simulink model "Torque_Control_ETR07"  (R2017b)
settings: Solver=FixedStepAuto  StartTime=0.0  StopTime=10.0  RelTol=1e-3
libraries: simulink x15
(part 3 of 5)

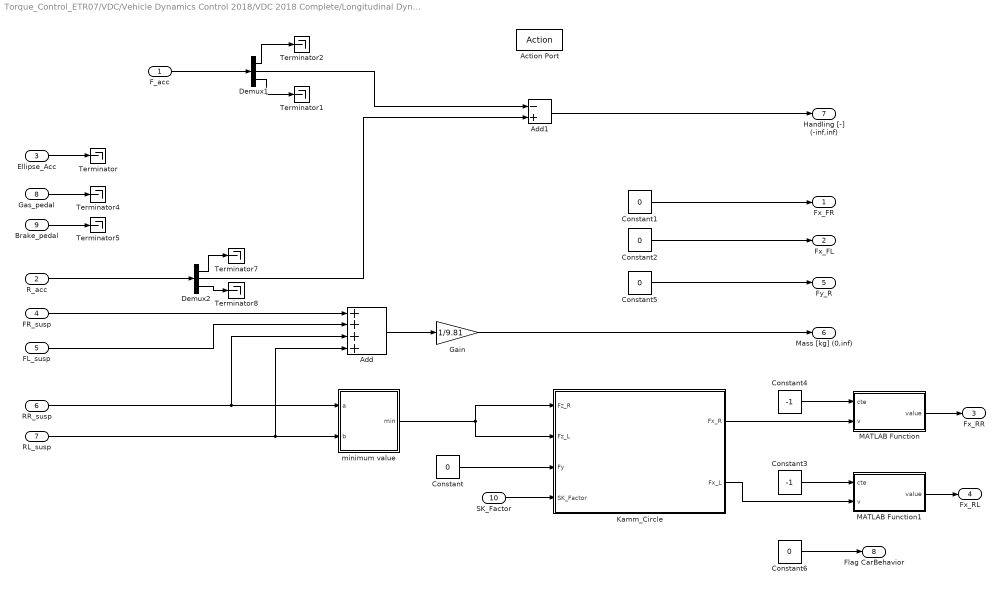
== system Torque_Control_ETR07/VDC/Vehicle Dynamics Control 2018/VDC 2018 Complete/Longitudinal Dynamics ==
  F_acc : Inport
  R_acc : Inport  Port=2
  Ellipse_Acc : Inport  Port=3
  FR_susp : Inport  Port=4
  FL_susp : Inport  Port=5
  RR_susp : Inport  Port=6
  RL_susp : Inport  Port=7
  Gas_pedal : Inport  Port=8
  Brake_pedal : Inport  Port=9
  SK_Factor : Inport  Port=10
  Action Port : ActionPort  ActionType=then
  Add : Sum  Inputs=++++
  Add1 : Sum  Inputs=-+
  Constant{,1..2,5..6} (5 alike) : Constant  Value=0
  Constant3 : Constant  Value=-1
  Constant4 : Constant  Value=-1
  Demux1 : Demux  Outputs=3
  Demux2 : Demux  Outputs=3
  Gain : Gain  Gain=1/9.81
  Kamm_Circle : Subsystem
  MATLAB Function : MATLAB Function  TreatAsAtomicUnit=on
  MATLAB Function1 : MATLAB Function  TreatAsAtomicUnit=on
  Terminator{,1..2,4..5,7..8} (7 alike) : Terminator
  minimum value : MATLAB Function  TreatAsAtomicUnit=on
  Fx_FR : Outport
  Fx_FL : Outport  Port=2
  "Fx_RR " : Outport  Port=3
  "Fx_RL " : Outport  Port=4
  Fy_R : Outport  Port=5
  Mass [kg] (0,inf) : Outport  Port=6
  Handling [-] (-inf,inf) : Outport  Port=7
  Flag CarBehavior : Outport  Port=8
  wires:
  Gas_pedal/1 -> Terminator4/1
  Brake_pedal/1 -> Terminator5/1
  Constant2/1 -> Fx_FL/1
  Constant1/1 -> Fx_FR/1
  Constant/1 -> Kamm_Circle/3(Fy)
  SK_Factor/1 -> Kamm_Circle/4(SK_Factor)
  minimum value/1(min) -> Kamm_Circle/1(Fz_R), Kamm_Circle/2(Fz_L)
  Gain/1 -> Mass [kg] (0,inf)/1
  Add/1 -> Gain/1
  F_acc/1 -> Demux1/1
  Demux1/1 -> Terminator2/1
  Demux1/3 -> Terminator1/1
  Add1/1 -> Handling [-] (-inf,inf)/1
  Demux1/2 -> Add1/1
  Kamm_Circle/1(Fx_R) -> MATLAB Function/2(v)
  Kamm_Circle/2(Fx_L) -> MATLAB Function1/2(v)
  Constant5/1 -> Fy_R/1
  Constant4/1 -> MATLAB Function/1(cte)
  MATLAB Function/1(value) -> "Fx_RR "/1
  MATLAB Function1/1(value) -> "Fx_RL "/1
  Constant3/1 -> MATLAB Function1/1(cte)
  Constant6/1 -> Flag CarBehavior/1
  FR_susp/1 -> Add/1
  FL_susp/1 -> Add/2
  RR_susp/1 -> Add/3, minimum value/1(a)
  RL_susp/1 -> minimum value/2(b), Add/4
  Demux2/2 -> Add1/2
  Demux2/3 -> Terminator8/1
  Demux2/1 -> Terminator7/1
  R_acc/1 -> Demux2/1
  Ellipse_Acc/1 -> Terminator/1

== system Torque_Control_ETR07/VDC/Vehicle Dynamics Control 2018/VDC 2018 Complete/Optimization SKF & CKF ==
  RPM_INV1 : Inport
  RPM_INV2 : Inport  Port=2
  Steer_An : Inport  Port=3
  SKF_Initial : Inport  Port=4
  CKF_Initial : Inport  Port=5
  Cte_SKF : Inport  Port=6
  Cte_CKF : Inport  Port=7
  CKF_prev : DataStoreRead  DataStoreName=B
  Constant : Constant  Value=0
  Data Store Memory : DataStoreMemory  ReadBeforeWriteMsg=warning  WriteAfterWriteMsg=warning  WriteAfterReadMsg=warning  ShowAdditionalParam=off
  Data Store Memory1 : DataStoreMemory  DataStoreName=B  ReadBeforeWriteMsg=warning  WriteAfterWriteMsg=warning  WriteAfterReadMsg=warning  ShowAdditionalParam=off
  Data Store Write : DataStoreWrite
  Data Store Write1 : DataStoreWrite  DataStoreName=B
  Derivative : Derivative
  Display : Display
  Display1 : Display
  Display2 : Display
  MATLAB Function : MATLAB Function  TreatAsAtomicUnit=on
  Mux : Mux  Inputs=3
  "SKF_prev " : DataStoreRead
  Saturation : Saturate  UpperLimit=6000  LowerLimit=0
  Scope : Scope
  "Subsystem " : Subsystem
  Switch : Switch  Threshold=900
  SKF_act : Outport
  CKF_act : Outport  Port=2
  wires:
  SKF_Initial/1 -> "Subsystem "/3(SKF_Initial)
  CKF_prev/1 -> "Subsystem "/6("CKF_prev ")
  "Subsystem "/1("SKF_act ") -> SKF_act/1, Display1/1, Data Store Write/1  "SKF"
  Derivative/1 -> Switch/1, Switch/2, Saturation/1, Display/1, "Subsystem "/2(Derivative)  "alpha"
  "SKF_prev "/1 -> "Subsystem "/4(SKF_prev)
  "Subsystem "/2(CKF_act) -> CKF_act/1, Display2/1, Data Store Write1/1  "CKF"
  Cte_CKF/1 -> "Subsystem "/8(Cte_CKF)
  Steer_An/1 -> "Subsystem "/1(Steer_An)
  CKF_Initial/1 -> "Subsystem "/5("CKF_Initial ")
  Cte_SKF/1 -> "Subsystem "/7(Cte_SKF)
  MATLAB Function/1(RPM) -> Derivative/1  "w (rad/s)"
  Mux/1 -> Scope/1
  Saturation/1 -> Mux/2
  Switch/1 -> Mux/3
  Constant/1 -> Switch/3
  RPM_INV1/1 -> Mux/1, MATLAB Function/1(RPM_INV1)
  RPM_INV2/1 -> MATLAB Function/2(RPM_INV2)

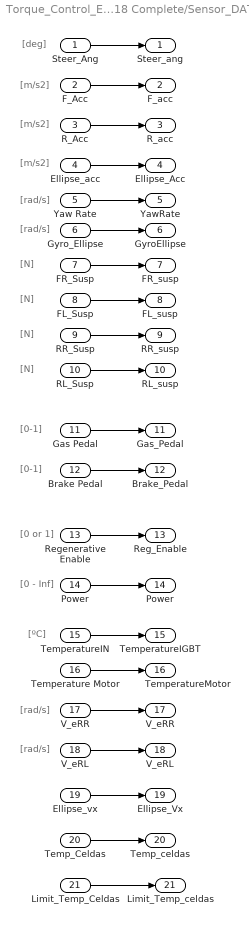
== system Torque_Control_ETR07/VDC/Vehicle Dynamics Control 2018/VDC 2018 Complete/Sensor_DATA ==
  note: [rad/s]
  note: [ºC]
  note: [m/s2]
  note: [m/s2]
  note: [deg]
  note: [N]
  note: [N]
  note: [N]
  note: [N]
  note: [0-1]
  note: [0-1]
  note: [0 or 1]
  note: [0 - Inf]
  note: [rad/s]
  note: [rad/s]
  note: [rad/s]
  note: [m/s2]
  Steer_Ang : Inport
  "F_Acc " : Inport  Port=2
  R_Acc : Inport  Port=3
  Ellipse_acc : Inport  Port=4
  Yaw Rate : Inport  Port=5
  Gyro_Ellipse : Inport  Port=6
  FR_Susp : Inport  Port=7
  FL_Susp : Inport  Port=8
  RR_Susp : Inport  Port=9
  RL_Susp : Inport  Port=10
  Gas Pedal : Inport  Port=11
  Brake Pedal : Inport  Port=12
  Regenerative Enable : Inport  Port=13
  "Power " : Inport  Port=14
  TemperatureIN : Inport  Port=15
  Temperature Motor : Inport  Port=16
  V_eRR : Inport  Port=17
  "V_eRL " : Inport  Port=18
  Ellipse_vx : Inport  Port=19
  Temp_Celdas : Inport  Port=20
  Limit_Temp_Celdas : Inport  Port=21
  Steer_ang : Outport
  F_acc : Outport  Port=2
  R_acc : Outport  Port=3
  Ellipse_Acc : Outport  Port=4
  YawRate : Outport  Port=5
  GyroEllipse : Outport  Port=6
  FR_susp : Outport  Port=7
  FL_susp : Outport  Port=8
  RR_susp : Outport  Port=9
  RL_susp : Outport  Port=10
  Gas_Pedal : Outport  Port=11
  Brake_Pedal : Outport  Port=12
  Reg_Enable : Outport  Port=13
  Power : Outport  Port=14
  TemperatureIGBT : Outport  Port=15
  TemperatureMotor : Outport  Port=16
  "V_eRR " : Outport  Port=17
  V_eRL : Outport  Port=18
  Ellipse_Vx : Outport  Port=19  VectorParamsAs1DForOutWhenUnconnected=on
  Temp_celdas : Outport  Port=20  VectorParamsAs1DForOutWhenUnconnected=on
  Limit_Temp_celdas : Outport  Port=21  VectorParamsAs1DForOutWhenUnconnected=on
  wires:
  RL_Susp/1 -> RL_susp/1
  RR_Susp/1 -> RR_susp/1
  FL_Susp/1 -> FL_susp/1
  FR_Susp/1 -> FR_susp/1
  Steer_Ang/1 -> Steer_ang/1
  R_Acc/1 -> R_acc/1
  "F_Acc "/1 -> F_acc/1
  Gas Pedal/1 -> Gas_Pedal/1
  Brake Pedal/1 -> Brake_Pedal/1
  Regenerative Enable/1 -> Reg_Enable/1
  "Power "/1 -> Power/1
  TemperatureIN/1 -> TemperatureIGBT/1
  "V_eRL "/1 -> V_eRL/1
  V_eRR/1 -> "V_eRR "/1
  Temperature Motor/1 -> TemperatureMotor/1
  Yaw Rate/1 -> YawRate/1
  Gyro_Ellipse/1 -> GyroEllipse/1
  Ellipse_acc/1 -> Ellipse_Acc/1
  Ellipse_vx/1 -> Ellipse_Vx/1
  Temp_Celdas/1 -> Temp_celdas/1
  Limit_Temp_Celdas/1 -> Limit_Temp_celdas/1

== system Torque_Control_ETR07/VDC/Vehicle Dynamics Control 2018/VDC 2018 Complete/Wheel_to_engine ==
  "Fx_FR " : Inport
  "Fx_FL " : Inport  Port=2
  "Fx_RR " : Inport  Port=3
  "Fx_RL " : Inport  Port=4
  Re : Inport  Port=5
  RT : Inport  Port=6
  Add : Sum  Inputs=+-
  Constant : Constant  Value=0
  Constant1 : Constant  Value=0
  Fx_to_engineTqRL : Subsystem
  Fx_to_engineTqRR : Subsystem
  MATLAB Function1 : MATLAB Function  TreatAsAtomicUnit=on
  MATLAB Function2 : MATLAB Function  TreatAsAtomicUnit=on
  Tq_diff : Outport  VectorParamsAs1DForOutWhenUnconnected=on
  Tq_FR : Outport  Port=2
  Tq_FL : Outport  Port=3
  Tq_RR : Outport  Port=4
  Tq_RL : Outport  Port=5
  wires:
  Fx_to_engineTqRR/1(Tq) -> Add/1, Tq_RR/1
  Fx_to_engineTqRL/1(Tq) -> Tq_RL/1, Add/2
  "Fx_FR "/1 -> Tq_FR/1
  "Fx_FL "/1 -> Tq_FL/1
  Re/1 -> Fx_to_engineTqRR/2(Re), Fx_to_engineTqRL/2(Re)
  RT/1 -> Fx_to_engineTqRR/3(RT), Fx_to_engineTqRL/3(RT)
  "Fx_RL "/1 -> MATLAB Function2/2(v)
  "Fx_RR "/1 -> MATLAB Function1/2(v)
  MATLAB Function2/1(value) -> Fx_to_engineTqRL/1(Fx)
  MATLAB Function1/1(value) -> Fx_to_engineTqRR/1(Fx)
  Constant1/1 -> MATLAB Function1/1(cte)
  Constant/1 -> MATLAB Function2/1(cte)
  Add/1 -> Tq_diff/1

== system Torque_Control_ETR07/VDC/Vehicle Dynamics Control 2018/VDC 2018 without Longitudinal/Constraints ==
  Tq_FRin : Inport
  Tq_FLin : Inport  Port=2
  Tq_RR_wc : Inport  Port=3
  "Tq_RL_wc " : Inport  Port=4
  "Trans_max_static " : Inport  Port=5
  Trans_max_dynamic : Inport  Port=6
  Power : Inport  Port=7
  Power_limit : Inport  Port=8
  ReductionCte_Power : Inport  Port=9
  ReductionCte_Temperature : Inport  Port=10
  TemperatureIGBT : Inport  Port=11
  TemperatureI_limit_Motor : Inport  Port=12
  TemperatureIMotor : Inport  Port=13
  Temperature_limit_IGBT : Inport  Port=14
  V_eRR : Inport  Port=15
  V_eRL : Inport  Port=16
  Tq_max : Inport  Port=17
  MaxRegTorque : Inport  Port=18
  Bp : Inport  Port=19
  Reg_enable : Inport  Port=20
  Temp_celdas : Inport  Port=21
  Limit_Temp_Celdas : Inport  Port=22
  Acelerating and braking without Regenerative : Subsystem  TreatAsAtomicUnit=on
  Braking with Regenerative : Subsystem  TreatAsAtomicUnit=on
  Constant : Constant  Value=0
  Constant1 : Constant  Value=0
  If : If  NumInputs=2  IfExpression=u2 == 1 & u1 > 0
  Merge1 : Merge
  Merge2 : Merge
  Tq_FRout : Outport
  "Tq_FLout " : Outport  Port=2
  Tq_RRout : Outport  Port=3
  Tq_RLout : Outport  Port=4
  wires:
  Constant1/1 -> "Tq_FLout "/1
  Constant/1 -> Tq_FRout/1
  Tq_RR_wc/1 -> Acelerating and braking without Regenerative/8(Tq_RR), Braking with Regenerative/2(Tq_RR_wc)
  "Tq_RL_wc "/1 -> Braking with Regenerative/3(Tq_RL_wc), Acelerating and braking without Regenerative/9(Tq_RL)
  Tq_max/1 -> Acelerating and braking without Regenerative/1(Tq_max)
  V_eRL/1 -> Acelerating and braking without Regenerative/3(V_eRL)
  Trans_max_dynamic/1 -> Acelerating and braking without Regenerative/4(Trans_max_dynamic)
  "Trans_max_static "/1 -> Acelerating and braking without Regenerative/5(Trans_max_static)
  Merge2/1 -> Tq_RLout/1
  Merge1/1 -> Tq_RRout/1
  Bp/1 -> If/1
  Reg_enable/1 -> If/2
  V_eRR/1 -> Acelerating and braking without Regenerative/2(V_eRR)
  If/1 -> Braking with Regenerative/Action
  If/2 -> Acelerating and braking without Regenerative/Action
  MaxRegTorque/1 -> Braking with Regenerative/1(MaxRegTorque)
  Tq_FRin/1 -> Acelerating and braking without Regenerative/6(Tq_FR)
  Tq_FLin/1 -> Acelerating and braking without Regenerative/7(Tq_FL)
  ReductionCte_Temperature/1 -> Acelerating and braking without Regenerative/18(ReductionCte_Temperature1)
  ReductionCte_Power/1 -> Acelerating and braking without Regenerative/19(ReductionCte_Power1)
  TemperatureIGBT/1 -> Acelerating and braking without Regenerative/13(Temperature_IGBT)
  Temperature_limit_IGBT/1 -> Acelerating and braking without Regenerative/12(Temperature_limit_IGBT1)
  Power/1 -> Acelerating and braking without Regenerative/11(Power1)
  Power_limit/1 -> Acelerating and braking without Regenerative/10(Power_limit1)
  Acelerating and braking without Regenerative/2(TQ_RL) -> Merge2/1
  Acelerating and braking without Regenerative/1(TQ_RR) -> Merge1/1
  Braking with Regenerative/1(TQ_RR) -> Merge1/2
  Braking with Regenerative/2(TQ_RL) -> Merge2/2
  TemperatureI_limit_Motor/1 -> Acelerating and braking without Regenerative/14(Temperature_limit_Motor)
  TemperatureIMotor/1 -> Acelerating and braking without Regenerative/15(Temperature_Motor)
  Temp_celdas/1 -> Acelerating and braking without Regenerative/16(Temp_Celdas)
  Limit_Temp_Celdas/1 -> Acelerating and braking without Regenerative/17(Lim_Temp_Celdas)

== system Torque_Control_ETR07/VDC/Vehicle Dynamics Control 2018/VDC 2018 without Longitudinal/Driver // CarBehaviours ==
  Tq_FRin : Inport
  Tq_FLin : Inport  Port=2
  Tq_RRin : Inport  Port=3
  "Tq_RLin " : Inport  Port=4
  Bp : Inport  Port=5
  Ap : Inport  Port=6
  Reg_enable : Inport  Port=7
  Ap_Sat_up : Inport  Port=8
  Ap_Sat_down : Inport  Port=9
  Accelerating : Subsystem  TreatAsAtomicUnit=on
  Braking Conditions : If  NumInputs=3  IfExpression=u1>0 & u2==0 & u3==1  ElseIfExpressions=u1>0 & u2==0 & u3==0, u1==0 & u2==0
  Constant : Constant  Value=0
  Constant1 : Constant  Value=0
  Inertia Braking : Subsystem  TreatAsAtomicUnit=on
  Mech_Braking : Subsystem  TreatAsAtomicUnit=on
  Merge : Merge  Inputs=4
  Merge1 : Merge  Inputs=4
  Regenerative+Mech Braking : Subsystem  TreatAsAtomicUnit=on
  Terminator : Terminator
  Terminator1 : Terminator
  Tq_FRout : Outport
  "Tq_FLout " : Outport  Port=2
  Tq_RRout : Outport  Port=3
  Tq_RLout : Outport  Port=4
  out_Throttle : Outport  Port=5
  wires:
  Constant1/1 -> "Tq_FLout "/1
  Constant/1 -> Tq_FRout/1
  Tq_FLin/1 -> Terminator1/1
  Tq_FRin/1 -> Terminator/1
  Merge/1 -> Tq_RRout/1
  Merge1/1 -> Tq_RLout/1
  Bp/1 -> Braking Conditions/1
  Ap/1 -> Accelerating/1(Ap), Braking Conditions/2
  Regenerative+Mech Braking/1("Tq_RR ") -> Merge/1
  Mech_Braking/1("Tq_RR ") -> Merge/2
  Inertia Braking/1("Tq_RR ") -> Merge/3
  Accelerating/1("Tq_RR ") -> Merge/4
  Regenerative+Mech Braking/2(Tq_RL) -> Merge1/1
  Mech_Braking/2(Tq_RL) -> Merge1/2
  Inertia Braking/2(Tq_RL) -> Merge1/3
  Accelerating/2(Tq_RL) -> Merge1/4
  Braking Conditions/1 -> Regenerative+Mech Braking/Action
  Braking Conditions/2 -> Mech_Braking/Action
  Braking Conditions/3 -> Inertia Braking/Action
  Braking Conditions/4 -> Accelerating/Action
  Tq_RRin/1 -> Regenerative+Mech Braking/1(RegTq_RR), Accelerating/4(Tq_RR)
  "Tq_RLin "/1 -> Regenerative+Mech Braking/2(RegTq_RL), Accelerating/5("Tq_RL ")
  Ap_Sat_up/1 -> Accelerating/2("Ap_Sat_up ")
  Ap_Sat_down/1 -> Accelerating/3(Ap_Sat_down)
  Reg_enable/1 -> Braking Conditions/3
  Accelerating/3(Out_Throttle) -> out_Throttle/1

== system Torque_Control_ETR07/VDC/Vehicle Dynamics Control 2018/VDC 2018 without Longitudinal/In_Numbers ==
  C-Kamm_Factor : Inport
  Max Regen Torque [Nm] : Inport  Port=2
  Limit Power [kW] : Inport  Port=3
  Limit Temperature IGBT [ºC] : Inport  Port=4
  Limit Temperature Motor [ºC] : Inport  Port=5
  Reduction Power [0-1] : Inport  Port=6
  Reduction Temperature [0-1] : Inport  Port=7
  Steering Saturation (per site) [deg] : Inport  Port=8
  Ap_Sat_Down [-] : Inport  Port=9
  Ap_Sat_Up [-] : Inport  Port=10
  3% difference : Gain  Gain=0.97
  Effective Rolling Radius[inch] : Constant  Value=13
  Engine+Inverter Performance [-] : Constant  Value=0.8
  Maximum Torque per engine [Nm] : Constant  Value=140
  Maximum Transmission Torque Dynamic [Nm] : Constant  Value=140
  Maximum Transmission Torque Static [Nm] : Constant  Value=130
  Transmision Ratio[-] : Constant  Value=4
  inch to m : Gain  Gain=0.0254
  Steer_Sat [deg] : Outport
  Tq_Max [Nm] : Outport  Port=2
  Cornering Kamm_Factor [0-2] : Outport  Port=3
  Transmision_Ratio[-] : Outport  Port=4
  Effective Rolling Radius[m] : Outport  Port=5
  Ap_Sat_down[-] : Outport  Port=6
  Ap_Sat_up[-] : Outport  Port=7
  Engine+Inverter Performance[-] : Outport  Port=8
  Trans_max _static[Nm] : Outport  Port=9
  Trans_max_dynamic [Nm] : Outport  Port=10
  "Power limit [KW] " : Outport  Port=11
  Temperature limit IGBT [ºC] : Outport  Port=12
  Temperature limit Motor [ºC] : Outport  Port=13
  Reduction Power (0-1) : Outport  Port=14
  Reduction Temperature (0-1) : Outport  Port=15
  MaxRegTorque [Nm] : Outport  Port=16
  wires:
  Maximum Torque per engine [Nm]/1 -> Tq_Max [Nm]/1
  Transmision Ratio[-]/1 -> Transmision_Ratio[-]/1
  Effective Rolling Radius[inch]/1 -> inch to m/1
  Maximum Transmission Torque Static [Nm]/1 -> Trans_max _static[Nm]/1
  Maximum Transmission Torque Dynamic [Nm]/1 -> Trans_max_dynamic [Nm]/1
  inch to m/1 -> 3% difference/1
  3% difference/1 -> Effective Rolling Radius[m]/1
  Engine+Inverter Performance [-]/1 -> Engine+Inverter Performance[-]/1
  Max Regen Torque [Nm]/1 -> MaxRegTorque [Nm]/1
  Limit Power [kW]/1 -> "Power limit [KW] "/1
  Limit Temperature IGBT [ºC]/1 -> Temperature limit IGBT [ºC]/1
  Reduction Power [0-1]/1 -> Reduction Power (0-1)/1
  C-Kamm_Factor/1 -> Cornering Kamm_Factor [0-2]/1
  Steering Saturation (per site) [deg]/1 -> Steer_Sat [deg]/1
  Ap_Sat_Up [-]/1 -> Ap_Sat_up[-]/1
  Ap_Sat_Down [-]/1 -> Ap_Sat_down[-]/1
  Reduction Temperature [0-1]/1 -> Reduction Temperature (0-1)/1
  Limit Temperature Motor [ºC]/1 -> Temperature limit Motor [ºC]/1

== system Torque_Control_ETR07/VDC/Vehicle Dynamics Control 2018/VDC 2018 without Longitudinal/Kamm Circle Lateral ==
  "N_FR " : Inport
  N_FL : Inport  Port=2
  N_RR : Inport  Port=3
  N_RL : Inport  Port=4
  Fy : Inport  Port=5
  CK_Factor : Inport  Port=6
  Constant : Constant  Value=-1
  Constant1 : Constant  Value=-1
  Kamm_Circle LatD : MATLAB Function  TreatAsAtomicUnit=on
  MATLAB Function1 : MATLAB Function  TreatAsAtomicUnit=on
  MATLAB Function2 : MATLAB Function  TreatAsAtomicUnit=on
  Product : Product
  Product1 : Product
  Fx_FR : Outport
  Fx_FL : Outport  Port=2
  "Fx_RR " : Outport  Port=3
  "Fx_RL " : Outport  Port=4
  wires:
  N_FL/1 -> Fx_FL/1
  "N_FR "/1 -> Fx_FR/1
  N_RL/1 -> Kamm_Circle LatD/2(Fz_L)
  Fy/1 -> Kamm_Circle LatD/3(Fy)
  N_RR/1 -> Kamm_Circle LatD/1(Fz_R)
  Kamm_Circle LatD/1(Fx_R) -> Product/1
  Kamm_Circle LatD/2(Fx_L) -> Product1/1
  CK_Factor/1 -> Product/2, Product1/2
  Product1/1 -> MATLAB Function1/2(v)
  Product/1 -> MATLAB Function2/2(v)
  Constant1/1 -> MATLAB Function2/1(cte)
  Constant/1 -> MATLAB Function1/1(cte)
  MATLAB Function2/1(value) -> "Fx_RR "/1
  MATLAB Function1/1(value) -> "Fx_RL "/1

== system Torque_Control_ETR07/VDC/Vehicle Dynamics Control 2018/VDC 2018 without Longitudinal/Lateral Dynamics ==
  F_acc : Inport
  R_acc : Inport  Port=2
  FR_susp : Inport  Port=3
  FL_susp : Inport  Port=4
  RR_susp : Inport  Port=5
  RL_susp : Inport  Port=6
  Gas_pedal : Inport  Port=7
  Brake_pedal : Inport  Port=8
  Ellipse_acc : Inport  Port=9
  Constant1 : Constant  Value=0
  Constant2 : Constant  Value=0
  Demux : Demux  Outputs=3
  Demux1 : Demux  Outputs=3
  Fy per wheel : Gain  Gain=1/2
  Gravity : Gain  Gain=1/9.81
  Gravity1 : Gain  Gain=1/9.81
  Product : Product
  Sum : Sum  Inputs=++++
  Sum1 : Sum
  Sum2 : Sum  Inputs=+-
  Terminator{,1..6} (7 alike) : Terminator
  N_FR : Outport
  "N_FL " : Outport  Port=2
  "N_RR " : Outport  Port=3
  N_RL : Outport  Port=4
  Fy_R : Outport  Port=5
  Mass [kg] (0,inf) : Outport  Port=6
  Handling [-] (-inf,inf) : Outport  Port=7
  wires:
  Constant2/1 -> "N_FL "/1
  Constant1/1 -> N_FR/1
  F_acc/1 -> Demux1/1
  Gas_pedal/1 -> Terminator4/1
  Brake_pedal/1 -> Terminator5/1
  Demux/2 -> Sum2/2, Product/1
  Demux/1 -> Terminator6/1
  Demux/3 -> Terminator3/1
  Product/1 -> Fy per wheel/1  "Fy per axe"
  Fy per wheel/1 -> Fy_R/1
  Gravity1/1 -> Product/2
  Sum/1 -> Gravity/1
  Sum1/1 -> Gravity1/1
  Gravity/1 -> Mass [kg] (0,inf)/1  "Mass [kg]"
  Demux1/1 -> Terminator1/1
  Demux1/3 -> Terminator2/1
  Demux1/2 -> Sum2/1
  Sum2/1 -> Handling [-] (-inf,inf)/1
  RL_susp/1 -> N_RL/1, Sum1/2, Sum/4
  RR_susp/1 -> Sum1/1, "N_RR "/1, Sum/3
  FL_susp/1 -> Sum/2
  FR_susp/1 -> Sum/1
  R_acc/1 -> Demux/1
  Ellipse_acc/1 -> Terminator/1

== system Torque_Control_ETR07/VDC/Vehicle Dynamics Control 2018/VDC 2018 without Longitudinal/Optimization SKF & CKF ==
  RPM_INV1 : Inport
  RPM_INV2 : Inport  Port=2
  CKF_Initial : Inport  Port=3
  Cte_CKF : Inport  Port=4
  CKF_prev : DataStoreRead  DataStoreName=B
  Data Store Memory1 : DataStoreMemory  DataStoreName=B  ReadBeforeWriteMsg=warning  WriteAfterWriteMsg=warning  WriteAfterReadMsg=warning  ShowAdditionalParam=off
  Data Store Write1 : DataStoreWrite  DataStoreName=B
  Derivative : Derivative
  MATLAB Function : MATLAB Function  TreatAsAtomicUnit=on
  "Subsystem " : Subsystem
  CKF_act : Outport
  wires:
  CKF_prev/1 -> "Subsystem "/3("CKF_prev ")
  Derivative/1 -> "Subsystem "/1(Derivative)  "alpha"
  MATLAB Function/1(RPM) -> Derivative/1  "w (rad/s)"
  "Subsystem "/1(CKF_act) -> Data Store Write1/1, CKF_act/1  "CKF"
  Cte_CKF/1 -> "Subsystem "/4(Cte_CKF)
  CKF_Initial/1 -> "Subsystem "/2("CKF_Initial ")
  RPM_INV1/1 -> MATLAB Function/1(RPM_INV1)
  RPM_INV2/1 -> MATLAB Function/2(RPM_INV2)

== system Torque_Control_ETR07/VDC/Vehicle Dynamics Control 2018/VDC 2018 without Longitudinal/Sensor_DATA ==
  note: [ºC]
  note: [m/s2]
  note: [m/s2]
  note: [deg]
  note: [N]
  note: [N]
  note: [N]
  note: [N]
  note: [0-1]
  note: [0-1]
  note: [0 or 1]
  note: [0 - Inf]
  note: [rad/s]
  note: [rad/s]
  Steer_Ang : Inport
  "F_Acc " : Inport  Port=2
  R_Acc : Inport  Port=3
  FR_Susp : Inport  Port=4
  FL_Susp : Inport  Port=5
  RR_Susp : Inport  Port=6
  RL_Susp : Inport  Port=7
  Gas Pedal : Inport  Port=8
  Brake Pedal : Inport  Port=9
  Regenerative Enable : Inport  Port=10
  "Power " : Inport  Port=11
  TemperatureIGBT : Inport  Port=12
  TemperatureMotor : Inport  Port=13
  V_eRR : Inport  Port=14
  "V_eRL " : Inport  Port=15
  Ellipse_acc_ax_ay_az : Inport  Port=16
  Temp_Celdas : Inport  Port=17
  Lim_Temp_Celdas : Inport  Port=18
  Steer_ang : Outport
  F_acc : Outport  Port=2
  R_acc : Outport  Port=3
  FR_susp : Outport  Port=4
  FL_susp : Outport  Port=5
  RR_susp : Outport  Port=6
  RL_susp : Outport  Port=7
  Gas_Pedal : Outport  Port=8
  Brake_Pedal : Outport  Port=9
  Reg_Enable : Outport  Port=10
  Power : Outport  Port=11
  Temperature IGBT : Outport  Port=12
  Temperature Motor : Outport  Port=13
  "V_eRR " : Outport  Port=14
  V_eRL : Outport  Port=15
  Ellipse_acc : Outport  Port=16
  temp_celdas : Outport  Port=17  VectorParamsAs1DForOutWhenUnconnected=on
  Lim_temp_celdas : Outport  Port=18  VectorParamsAs1DForOutWhenUnconnected=on
  wires:
  RL_Susp/1 -> RL_susp/1
  RR_Susp/1 -> RR_susp/1
  FL_Susp/1 -> FL_susp/1
  FR_Susp/1 -> FR_susp/1
  Steer_Ang/1 -> Steer_ang/1
  R_Acc/1 -> R_acc/1
  "F_Acc "/1 -> F_acc/1
  Gas Pedal/1 -> Gas_Pedal/1
  Brake Pedal/1 -> Brake_Pedal/1
  Regenerative Enable/1 -> Reg_Enable/1
  "Power "/1 -> Power/1
  TemperatureIGBT/1 -> Temperature IGBT/1
  "V_eRL "/1 -> V_eRL/1
  V_eRR/1 -> "V_eRR "/1
  TemperatureMotor/1 -> Temperature Motor/1
  Ellipse_acc_ax_ay_az/1 -> Ellipse_acc/1
  Temp_Celdas/1 -> temp_celdas/1
  Lim_Temp_Celdas/1 -> Lim_temp_celdas/1

== system Torque_Control_ETR07/VDC/Vehicle Dynamics Control 2018/VDC 2018 without Longitudinal/Wheel_to_engine ==
  "Fx_FR " : Inport
  "Fx_FL " : Inport  Port=2
  "Fx_RR " : Inport  Port=3
  "Fx_RL " : Inport  Port=4
  Re : Inport  Port=5
  RT : Inport  Port=6
  Constant : Constant  Value=0
  Constant1 : Constant  Value=0
  Fx_to_engineTqRL : Subsystem
  Fx_to_engineTqRR : Subsystem
  MATLAB Function1 : MATLAB Function  TreatAsAtomicUnit=on
  MATLAB Function2 : MATLAB Function  TreatAsAtomicUnit=on
  Tq_FR : Outport
  Tq_FL : Outport  Port=2
  Tq_RR : Outport  Port=3
  Tq_RL : Outport  Port=4
  wires:
  Fx_to_engineTqRR/1(Tq) -> Tq_RR/1
  Fx_to_engineTqRL/1(Tq) -> Tq_RL/1
  "Fx_FR "/1 -> Tq_FR/1
  "Fx_FL "/1 -> Tq_FL/1
  Re/1 -> Fx_to_engineTqRR/2(Re), Fx_to_engineTqRL/2(Re)
  RT/1 -> Fx_to_engineTqRR/3(RT), Fx_to_engineTqRL/3(RT)
  "Fx_RR "/1 -> MATLAB Function2/2(v)
  "Fx_RL "/1 -> MATLAB Function1/2(v)
  MATLAB Function2/1(value) -> Fx_to_engineTqRR/1(Fx)
  Constant/1 -> MATLAB Function2/1(cte)
  Constant1/1 -> MATLAB Function1/1(cte)
  MATLAB Function1/1(value) -> Fx_to_engineTqRL/1(Fx)

== system Torque_Control_ETR07/VDC/Vehicle Dynamics Control 2018/Steering TV 2017 with TC/Constraints/Control de Potencia  ==
  Tq_RR : Inport
  Tq_RL : Inport  Port=2
  ReductionCte : Inport  Port=3
  Action Port : ActionPort  ActionType=elseif
  Add : Sum  Inputs=+-
  Add1 : Sum  Inputs=+-
  Product : Product
  Product1 : Product
  Tq_RR_out : Outport
  Tq_RL_out : Outport  Port=2
  wires:
  Tq_RR/1 -> Product/1, Add/1
  Tq_RL/1 -> Product1/1, Add1/1
  ReductionCte/1 -> Product/2, Product1/2
  Product1/1 -> Add1/2
  Product/1 -> Add/2
  Add1/1 -> Tq_RL_out/1
  Add/1 -> Tq_RR_out/1

== system Torque_Control_ETR07/VDC/Vehicle Dynamics Control 2018/Steering TV 2017 with TC/Constraints/Control de Temperatura ==
  Tq_RR : Inport
  Tq_RL : Inport  Port=2
  ReductionCte : Inport  Port=3
  Action Port : ActionPort  ActionType=then
  Add : Sum  Inputs=+-
  Add1 : Sum  Inputs=+-
  Product : Product
  Product1 : Product
  Tq_RR_out : Outport
  Tq_RL_out : Outport  Port=2
  wires:
  Product/1 -> Add/2
  Product1/1 -> Add1/2
  Add1/1 -> Tq_RL_out/1
  Tq_RR/1 -> Add/1, Product/1
  Tq_RL/1 -> Add1/1, Product1/1
  ReductionCte/1 -> Product1/2, Product/2
  Add/1 -> Tq_RR_out/1

== system Torque_Control_ETR07/VDC/Vehicle Dynamics Control 2018/Steering TV 2017 with TC/Constraints/else ==
  Tq_RR : Inport
  Tq_RL : Inport  Port=2
  Action Port : ActionPort  ActionType=else
  Tq_RR_out : Outport
  Tq_RL_out : Outport  Port=2
  wires:
  Tq_RR/1 -> Tq_RR_out/1
  Tq_RL/1 -> Tq_RL_out/1

== system Torque_Control_ETR07/VDC/Vehicle Dynamics Control 2018/Steering TV 2017 with TC/Optimization SKF & CKF/Subsystem  ==
  Steer_An : Inport
  Derivative : Inport  Port=2
  SKF_Initial : Inport  Port=3
  SKF_prev : Inport  Port=4
  "CKF_Initial " : Inport  Port=5
  "CKF_prev " : Inport  Port=6
  Cte_SKF : Inport  Port=7
  Cte_CKF : Inport  Port=8
  CKF : Subsystem
  MATLAB Function1 : MATLAB Function  TreatAsAtomicUnit=on
  SKF : Subsystem
  SKF or CKF : If  IfExpression=-10 < u1 & u1 < 10
  Steering Wheel Maximum Angle : Constant  Value=100
  "SKF_act " : Outport
  CKF_act : Outport  Port=2
  wires:
  MATLAB Function1/1(value) -> SKF or CKF/1
  Steering Wheel Maximum Angle/1 -> MATLAB Function1/1(cte)
  Steer_An/1 -> MATLAB Function1/2(v)
  SKF/1(SKF_act) -> "SKF_act "/1
  CKF/1("CKF_act ") -> CKF_act/1
  SKF or CKF/1 -> SKF/Action
  SKF or CKF/2 -> CKF/Action
  "CKF_prev "/1 -> CKF/3("CKF_prev ")
  Derivative/1 -> CKF/1(Derivative), SKF/1(Derivative)
  SKF_Initial/1 -> SKF/2("SKF_Initial ")
  SKF_prev/1 -> SKF/3(SKF_prev)
  "CKF_Initial "/1 -> CKF/2(CKF_Initial)
  Cte_SKF/1 -> SKF/4(Cte_SKF)
  Cte_CKF/1 -> CKF/4(Cte_CKF)

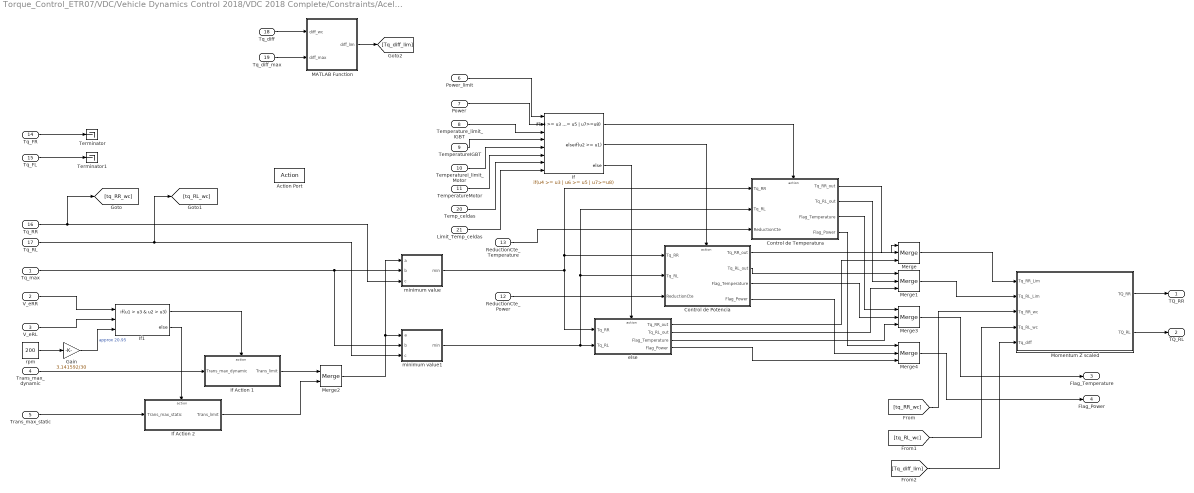
== system Torque_Control_ETR07/VDC/Vehicle Dynamics Control 2018/VDC 2018 Complete/Constraints/Acelerating and braking without Regenerative ==
  Tq_max : Inport
  V_eRR : Inport  Port=2
  V_eRL : Inport  Port=3
  Trans_max_dynamic : Inport  Port=4
  Trans_max_static : Inport  Port=5
  Power_limit : Inport  Port=6
  Power : Inport  Port=7
  Temperature_limit_IGBT : Inport  Port=8
  TemperatureIGBT : Inport  Port=9
  TemperatureI_limit_Motor : Inport  Port=10
  TemperatureMotor : Inport  Port=11
  ReductionCte_Power : Inport  Port=12
  ReductionCte_Temperature : Inport  Port=13
  Tq_FR : Inport  Port=14
  Tq_FL : Inport  Port=15
  Tq_RR : Inport  Port=16
  Tq_RL : Inport  Port=17
  Tq_diff : Inport  Port=18
  Tq_diff_max : Inport  Port=19
  Temp_celdas : Inport  Port=20
  Limit_Temp_celdas : Inport  Port=21
  Action Port : ActionPort  ActionType=else
  "Control de Potencia " : Subsystem  TreatAsAtomicUnit=on
  Control de Temperatura : Subsystem  TreatAsAtomicUnit=on
  Gain : Gain  Gain=3.141592/30
  If : If  NumInputs=8  IfExpression=u4 >= u3 | u6 >= u5 | u7>=u8  ElseIfExpressions=u2 >= u1
  If Action 1 : Subsystem  TreatAsAtomicUnit=on
  If Action 2 : Subsystem  TreatAsAtomicUnit=on
  If1 : If  NumInputs=3  IfExpression=u1 > u3 & u2 > u3
  MATLAB Function : MATLAB Function  TreatAsAtomicUnit=on
  Merge{,1,3..4} (4 alike) : Merge  Inputs=3
  Merge2 : Merge
  Momentum Z scaled : Subsystem
  Terminator : Terminator
  Terminator1 : Terminator
  else : Subsystem  TreatAsAtomicUnit=on
  minimum value : MATLAB Function  TreatAsAtomicUnit=on
  minimum value1 : MATLAB Function  TreatAsAtomicUnit=on
  rpm : Constant  Value=200
  TQ_RR : Outport
  TQ_RL : Outport  Port=2
  Flag_Temperature : Outport  Port=3
  Flag_Power : Outport  Port=4
  wires:
  If1/1 -> If Action 1/Action
  If Action 1/1(Trans_limit) -> Merge2/1
  Merge2/1 -> minimum value/1(a), minimum value1/1(a)
  Trans_max_dynamic/1 -> If Action 1/1(Trans_max_dynamic)
  If Action 2/1(Trans_limit) -> Merge2/2
  V_eRR/1 -> If1/1
  V_eRL/1 -> If1/2
  If1/2 -> If Action 2/Action
  Trans_max_static/1 -> If Action 2/1("Trans_max_static ")
  Tq_max/1 -> minimum value1/2(b), minimum value/2(b)
  rpm/1 -> Gain/1
  Gain/1 -> If1/3  "approx 20.95"
  Tq_FR/1 -> Terminator/1
  Tq_FL/1 -> Terminator1/1
  TemperatureIGBT/1 -> If/4
  ReductionCte_Power/1 -> "Control de Potencia "/3(ReductionCte)
  If/3 -> else/Action
  Power_limit/1 -> If/1
  Power/1 -> If/2
  Temperature_limit_IGBT/1 -> If/3
  minimum value/1(min) -> Control de Temperatura/1(Tq_RR), "Control de Potencia "/1(Tq_RR), else/1(Tq_RR)
  minimum value1/1(min) -> Control de Temperatura/2(Tq_RL), "Control de Potencia "/2(Tq_RL), else/2(Tq_RL)
  ReductionCte_Temperature/1 -> Control de Temperatura/3(ReductionCte)
  "Control de Potencia "/1(Tq_RR_out) -> Merge/1
  Control de Temperatura/1(Tq_RR_out) -> Merge/2
  else/1(Tq_RR_out) -> Merge/3
  "Control de Potencia "/2(Tq_RL_out) -> Merge1/1
  Control de Temperatura/2(Tq_RL_out) -> Merge1/2
  else/2(Tq_RL_out) -> Merge1/3
  If/1 -> Control de Temperatura/Action
  If/2 -> "Control de Potencia "/Action
  Tq_RR/1 -> [tq_RR_wc], minimum value/3(c)
  Tq_RL/1 -> [tq_RL_wc], minimum value1/3(c)
  Merge/1 -> Momentum Z scaled/1(Tq_RR_Lim)
  Merge1/1 -> Momentum Z scaled/2(Tq_RL_Lim)
  [tq_RR_wc] -> Momentum Z scaled/3(Tq_RR_wc)
  [tq_RL_wc] -> Momentum Z scaled/4(Tq_RL_wc)
  TemperatureI_limit_Motor/1 -> If/5
  TemperatureMotor/1 -> If/6
  Merge3/1 -> Flag_Temperature/1
  Merge4/1 -> Flag_Power/1
  Control de Temperatura/3(Flag_Temperature) -> Merge3/1
  Control de Temperatura/4(Flag_Power) -> Merge4/1
  "Control de Potencia "/3(Flag_Temperature) -> Merge3/2
  "Control de Potencia "/4(Flag_Power) -> Merge4/2
  else/3(Flag_Temperature) -> Merge3/3
  else/4(Flag_Power) -> Merge4/3
  Momentum Z scaled/1(TQ_RR) -> TQ_RR/1
  Momentum Z scaled/2(TQ_RL) -> TQ_RL/1
  Tq_diff/1 -> MATLAB Function/1(diff_wc)
  Tq_diff_max/1 -> MATLAB Function/2(diff_max)
  MATLAB Function/1(diff_lim) -> [Tq_diff_lim]
  [Tq_diff_lim] -> Momentum Z scaled/5(Tq_diff)
  Temp_celdas/1 -> If/7
  Limit_Temp_celdas/1 -> If/8

== system Torque_Control_ETR07/VDC/Vehicle Dynamics Control 2018/VDC 2018 Complete/Constraints/Braking with Regenerative ==
  MaxRegTorque : Inport
  Tq_RR_wc : Inport  Port=2
  Tq_RL_wc : Inport  Port=3
  Action Port : ActionPort  ActionType=then
  Gain : Gain  Gain=-1
  Gain1 : Gain  Gain=-1
  MATLAB Function : MATLAB Function  TreatAsAtomicUnit=on
  TQ_RR : Outport
  TQ_RL : Outport  Port=2
  wires:
  MATLAB Function/2(RegTq_RL) -> Gain1/1
  MATLAB Function/1(RegTq_RR) -> Gain/1
  Tq_RR_wc/1 -> MATLAB Function/2(Tq_RR)
  Tq_RL_wc/1 -> MATLAB Function/3(Tq_RL)
  MaxRegTorque/1 -> MATLAB Function/1(MaxRegenTq)
  Gain1/1 -> TQ_RL/1
  Gain/1 -> TQ_RR/1

== system Torque_Control_ETR07/VDC/Vehicle Dynamics Control 2018/VDC 2018 Complete/Driver // CarBehaviours/Accelerating ==
  Throttle : Inport
  Tq_RR : Inport  Port=2
  "Tq_RL " : Inport  Port=3
  Action Port : ActionPort  ActionType=else
  Product : Product
  Product1 : Product
  "Tq_RR " : Outport
  Tq_RL : Outport  Port=2
  Out_Throttle : Outport  Port=3
  wires:
  Product1/1 -> "Tq_RR "/1
  Product/1 -> Tq_RL/1
  Throttle/1 -> Out_Throttle/1, Product/1, Product1/1
  Tq_RR/1 -> Product1/2
  "Tq_RL "/1 -> Product/2

== system Torque_Control_ETR07/VDC/Vehicle Dynamics Control 2018/VDC 2018 Complete/Driver // CarBehaviours/Inertia Braking ==
  Action Port : ActionPort  ActionType=elseif
  Constant : Constant  Value=0
  Constant1 : Constant  Value=0
  "Tq_RR " : Outport
  Tq_RL : Outport  Port=2
  wires:
  Constant1/1 -> Tq_RL/1
  Constant/1 -> "Tq_RR "/1

== system Torque_Control_ETR07/VDC/Vehicle Dynamics Control 2018/VDC 2018 Complete/Driver // CarBehaviours/Mech_Braking ==
  Action Port : ActionPort  ActionType=elseif
  Constant : Constant  Value=0
  Constant1 : Constant  Value=0
  "Tq_RR " : Outport
  Tq_RL : Outport  Port=2
  wires:
  Constant1/1 -> Tq_RL/1
  Constant/1 -> "Tq_RR "/1

== system Torque_Control_ETR07/VDC/Vehicle Dynamics Control 2018/VDC 2018 Complete/Driver // CarBehaviours/Regenerative+Mech Braking ==
  RegTq_RR : Inport
  RegTq_RL : Inport  Port=2
  Action Port : ActionPort  ActionType=then
  "Tq_RR " : Outport
  Tq_RL : Outport  Port=2
  wires:
  RegTq_RR/1 -> "Tq_RR "/1
  RegTq_RL/1 -> Tq_RL/1

== system Torque_Control_ETR07/VDC/Vehicle Dynamics Control 2018/VDC 2018 Complete/Lateral Dynamics/Kamm_Circle ==
  Fz_R : Inport
  Fz_L : Inport  Port=2
  Fy : Inport  Port=3
  CK_Factor : Inport  Port=4
  Kamm_Circle LatD : MATLAB Function  TreatAsAtomicUnit=on
  Product1 : Product
  Product2 : Product
  Fx_R : Outport
  Fx_L : Outport  Port=2
  Fy_R [N] (0,inf) : Outport  Port=3
  wires:
  Kamm_Circle LatD/3(Fy_R) -> Fy_R [N] (0,inf)/1
  Fz_L/1 -> Kamm_Circle LatD/2(Fz_L)
  Fz_R/1 -> Kamm_Circle LatD/1(Fz_R)
  Fy/1 -> Kamm_Circle LatD/3(Fy)
  Kamm_Circle LatD/1(Fx_R) -> Product1/1
  Kamm_Circle LatD/2(Fx_L) -> Product2/1
  Product2/1 -> Fx_L/1
  CK_Factor/1 -> Product2/2, Product1/2
  Product1/1 -> Fx_R/1

== system Torque_Control_ETR07/VDC/Vehicle Dynamics Control 2018/VDC 2018 Complete/Lateral Dynamics/Tire Longitudinal Force Difference ==
  e : Inport
  Iz : Inport  Port=2
  dt : Inport  Port=3
  rt : Inport  Port=4
  " Momentum_Z to Longitudinal Force Difference" : Subsystem
  Momentum respect to Z-axis to correct the error : Subsystem
  Scope5 : Scope
  Scope6 : Scope
  Fx_diff : Outport
  wires:
  dt/1 -> Momentum respect to Z-axis to correct the error/3(Correction_Time [s])
  rt/1 -> " Momentum_Z to Longitudinal Force Difference"/2(RearTrackwidth [m])
  " Momentum_Z to Longitudinal Force Difference"/1(Fx_diff [N]) -> Fx_diff/1
  Iz/1 -> Momentum respect to Z-axis to correct the error/2(Iz [kg/m^3])
  Momentum respect to Z-axis to correct the error/1(Momentum_Z [Nm]) -> " Momentum_Z to Longitudinal Force Difference"/1("\tMomentumZ [Nm]"), Scope6/1
  e/1 -> Scope5/1, Momentum respect to Z-axis to correct the error/1(Yaw_error_[º/s])

== system Torque_Control_ETR07/VDC/Vehicle Dynamics Control 2018/VDC 2018 Complete/Lateral Dynamics/Yaw_Rate_Reference ==
  Steering_Angle : Inport
  F_vel_x : Inport  Port=2
  360/(2*pi) : Gain  Gain=360/(2*pi)
  360/(2pi) : Gain  Gain=360/(2*pi)
  Bicycle Model : MATLAB Function  TreatAsAtomicUnit=on
  Constant7 : Constant  Value=0.92
  Constant8 : Constant  Value=360
  Cornering_Stiffness_F[N/º] : Constant  Value=-700
  Cornering_Stiffness_R[N/º] : Constant  Value=-1000
  Divide : Product  Inputs=*/
  Gain{,1..4} (5 alike) : Gain  Gain=360/(2*pi)
  Scope1 : Scope  NumInputPorts=5
  Scope2 : Scope  NumInputPorts=2
  Scope3 : Scope
  Steering_Ratio [-] : Constant  Value=3.72
  Wheelbase [m] : Constant  Value=1.53
  Yaw_Rate : Outport
  wires:
  Gain4/1 -> Scope1/2
  Gain3/1 -> Scope1/3
  Gain2/1 -> Scope1/4
  Gain1/1 -> Scope1/1
  Gain/1 -> Scope1/5
  360/(2pi)/1 -> Bicycle Model/7(cr)
  Cornering_Stiffness_R[N/º]/1 -> 360/(2pi)/1
  360/(2*pi)/1 -> Bicycle Model/6(cf)
  Bicycle Model/2(beta) -> Gain2/1
  F_vel_x/1 -> Bicycle Model/2(vx)
  Bicycle Model/7(yf) -> Scope2/1
  Bicycle Model/3(alpha_f) -> Gain4/1
  Bicycle Model/6(radius) -> Scope3/1
  Cornering_Stiffness_F[N/º]/1 -> 360/(2*pi)/1
  Constant7/1 -> Bicycle Model/4(xCG)
  Bicycle Model/5(course) -> Gain/1
  Constant8/1 -> Bicycle Model/3(m)
  Bicycle Model/4(alpha_r) -> Gain3/1
  Steering_Ratio [-]/1 -> Divide/2
  Bicycle Model/1(r) -> Yaw_Rate/1
  Divide/1 -> Gain1/1, Bicycle Model/1(delta)
  Wheelbase [m]/1 -> Bicycle Model/5(L)
  Steering_Angle/1 -> Divide/1
  Bicycle Model/8(yr) -> Scope2/2

== system Torque_Control_ETR07/VDC/Vehicle Dynamics Control 2018/VDC 2018 Complete/Longitudinal Dynamics/Kamm_Circle ==
  Fz_R : Inport
  Fz_L : Inport  Port=2
  Fy : Inport  Port=3
  SK_Factor : Inport  Port=4
  Kamm_Circle LatD : MATLAB Function  TreatAsAtomicUnit=on
  Product : Product
  Product1 : Product
  Fx_R : Outport
  Fx_L : Outport  Port=2
  wires:
  Kamm_Circle LatD/1(Fx_R) -> Product/1
  Kamm_Circle LatD/2(Fx_L) -> Product1/1
  Fz_L/1 -> Kamm_Circle LatD/2(Fz_L)
  Fy/1 -> Kamm_Circle LatD/3(Fy)
  SK_Factor/1 -> Product/2, Product1/2
  Product/1 -> Fx_R/1
  Product1/1 -> Fx_L/1
  Fz_R/1 -> Kamm_Circle LatD/1(Fz_R)

== system Torque_Control_ETR07/VDC/Vehicle Dynamics Control 2018/VDC 2018 Complete/Optimization SKF & CKF/Subsystem  ==
  Steer_An : Inport
  Derivative : Inport  Port=2
  SKF_Initial : Inport  Port=3
  SKF_prev : Inport  Port=4
  "CKF_Initial " : Inport  Port=5
  "CKF_prev " : Inport  Port=6
  Cte_SKF : Inport  Port=7
  Cte_CKF : Inport  Port=8
  CKF : Subsystem
  MATLAB Function1 : MATLAB Function  TreatAsAtomicUnit=on
  SKF : Subsystem
  SKF or CKF : If  IfExpression=-10 < u1 & u1 < 10
  Steering Wheel Maximum Angle : Constant  Value=100
  "SKF_act " : Outport
  CKF_act : Outport  Port=2
  wires:
  MATLAB Function1/1(value) -> SKF or CKF/1
  Steering Wheel Maximum Angle/1 -> MATLAB Function1/1(cte)
  Steer_An/1 -> MATLAB Function1/2(v)
  SKF/1(SKF_act) -> "SKF_act "/1
  CKF/1("CKF_act ") -> CKF_act/1
  SKF or CKF/1 -> SKF/Action
  SKF or CKF/2 -> CKF/Action
  "CKF_prev "/1 -> CKF/3("CKF_prev ")
  Derivative/1 -> CKF/1(Derivative), SKF/1(Derivative)
  SKF_Initial/1 -> SKF/2("SKF_Initial ")
  SKF_prev/1 -> SKF/3(SKF_prev)
  "CKF_Initial "/1 -> CKF/2(CKF_Initial)
  Cte_SKF/1 -> SKF/4(Cte_SKF)
  Cte_CKF/1 -> CKF/4(Cte_CKF)

== system Torque_Control_ETR07/VDC/Vehicle Dynamics Control 2018/VDC 2018 Complete/Wheel_to_engine/Fx_to_engineTqRL ==
  Fx : Inport
  Re : Inport  Port=2
  RT : Inport  Port=3
  Divide : Product  Inputs=*/
  Product : Product
  Tq : Outport
  wires:
  Divide/1 -> Tq/1
  Product/1 -> Divide/1
  RT/1 -> Divide/2
  Fx/1 -> Product/1
  Re/1 -> Product/2

== system Torque_Control_ETR07/VDC/Vehicle Dynamics Control 2018/VDC 2018 Complete/Wheel_to_engine/Fx_to_engineTqRR ==
  Fx : Inport
  Re : Inport  Port=2
  RT : Inport  Port=3
  Divide : Product  Inputs=*/
  Product : Product
  Tq : Outport
  wires:
  Divide/1 -> Tq/1
  Product/1 -> Divide/1
  RT/1 -> Divide/2
  Fx/1 -> Product/1
  Re/1 -> Product/2

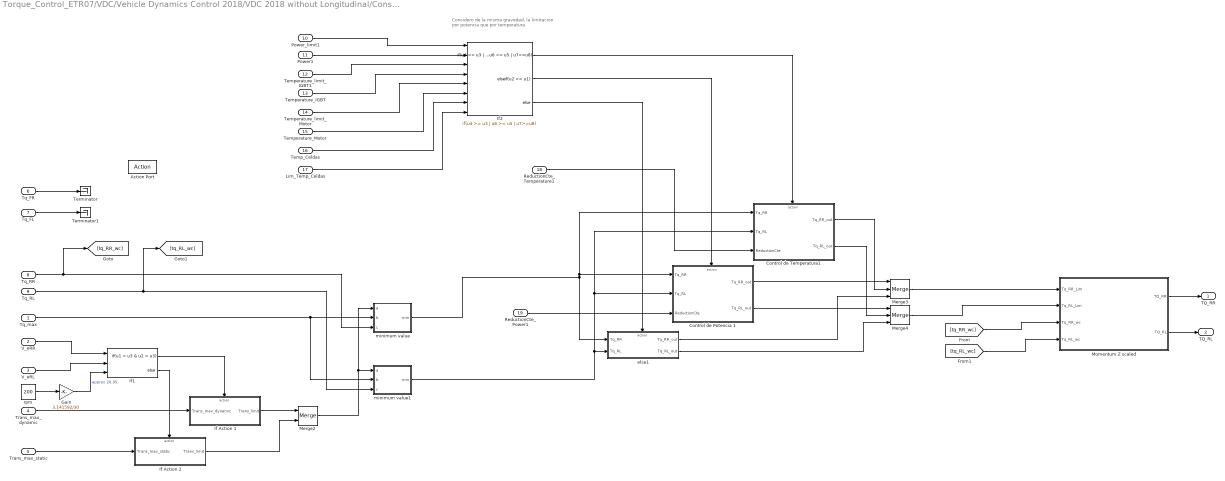
== system Torque_Control_ETR07/VDC/Vehicle Dynamics Control 2018/VDC 2018 without Longitudinal/Constraints/Acelerating and braking without Regenerative ==
  note: Considero de la misma gravedad,
      | la limitacion por potencia que por temperatura
  Tq_max : Inport
  V_eRR : Inport  Port=2
  V_eRL : Inport  Port=3
  Trans_max_dynamic : Inport  Port=4
  Trans_max_static : Inport  Port=5
  Tq_FR : Inport  Port=6
  Tq_FL : Inport  Port=7
  Tq_RR : Inport  Port=8
  Tq_RL : Inport  Port=9
  Power_limit1 : Inport  Port=10
  Power1 : Inport  Port=11
  Temperature_limit_IGBT1 : Inport  Port=12
  Temperature_IGBT : Inport  Port=13
  Temperature_limit_Motor : Inport  Port=14
  Temperature_Motor : Inport  Port=15
  Temp_Celdas : Inport  Port=16
  Lim_Temp_Celdas : Inport  Port=17
  ReductionCte_Temperature1 : Inport  Port=18
  ReductionCte_Power1 : Inport  Port=19
  Action Port : ActionPort  ActionType=else
  Control de Potencia 1 : Subsystem  TreatAsAtomicUnit=on
  Control de Temperatura1 : Subsystem  TreatAsAtomicUnit=on
  Gain : Gain  Gain=3.141592/30
  If Action 1 : Subsystem  TreatAsAtomicUnit=on
  If Action 2 : Subsystem  TreatAsAtomicUnit=on
  If1 : If  NumInputs=3  IfExpression=u1 > u3 & u2 > u3
  If2 : If  NumInputs=8  IfExpression=u4 >= u3 | u6 >= u5 | u7>=u8  ElseIfExpressions=u2 >= u1
  Merge2 : Merge
  Merge3 : Merge  Inputs=3
  Merge4 : Merge  Inputs=3
  Momentum Z scaled : Subsystem
  Terminator : Terminator
  Terminator1 : Terminator
  else1 : Subsystem  TreatAsAtomicUnit=on
  minimum value : MATLAB Function  TreatAsAtomicUnit=on
  minimum value1 : MATLAB Function  TreatAsAtomicUnit=on
  rpm : Constant  Value=200
  TQ_RR : Outport
  TQ_RL : Outport  Port=2
  wires:
  If1/1 -> If Action 1/Action
  If Action 1/1(Trans_limit) -> Merge2/1
  Merge2/1 -> minimum value/1(a), minimum value1/1(a)
  Trans_max_dynamic/1 -> If Action 1/1(Trans_max_dynamic)
  If Action 2/1(Trans_limit) -> Merge2/2
  V_eRR/1 -> If1/1
  V_eRL/1 -> If1/2
  If1/2 -> If Action 2/Action
  Trans_max_static/1 -> If Action 2/1("Trans_max_static ")
  Tq_max/1 -> minimum value1/2(b), minimum value/2(b)
  rpm/1 -> Gain/1
  Gain/1 -> If1/3  "approx 20.95"
  Tq_FR/1 -> Terminator/1
  Tq_FL/1 -> Terminator1/1
  Tq_RR/1 -> [tq_RR_wc], minimum value/3(c)
  Tq_RL/1 -> [tq_RL_wc], minimum value1/3(c)
  Merge3/1 -> Momentum Z scaled/1(Tq_RR_Lim)
  Merge4/1 -> Momentum Z scaled/2(Tq_RL_Lim)
  [tq_RR_wc] -> Momentum Z scaled/3(Tq_RR_wc)
  [tq_RL_wc] -> Momentum Z scaled/4(Tq_RL_wc)
  Momentum Z scaled/1(TQ_RR) -> TQ_RR/1
  Momentum Z scaled/2(TQ_RL) -> TQ_RL/1
  Temp_Celdas/1 -> If2/7
  Lim_Temp_Celdas/1 -> If2/8
  Control de Temperatura1/1(Tq_RR_out) -> Merge3/2
  Temperature_limit_Motor/1 -> If2/5
  Temperature_Motor/1 -> If2/6
  else1/1(Tq_RR_out) -> Merge3/3
  Control de Temperatura1/2(Tq_RL_out) -> Merge4/2
  If2/2 -> Control de Potencia 1/Action
  If2/3 -> else1/Action
  else1/2(Tq_RL_out) -> Merge4/3
  minimum value/1(min) -> Control de Temperatura1/1(Tq_RR), Control de Potencia 1/1(Tq_RR), else1/1(Tq_RR)
  Control de Potencia 1/1(Tq_RR_out) -> Merge3/1
  ReductionCte_Temperature1/1 -> Control de Temperatura1/3(ReductionCte)
  If2/1 -> Control de Temperatura1/Action
  Temperature_limit_IGBT1/1 -> If2/3
  Power1/1 -> If2/2
  ReductionCte_Power1/1 -> Control de Potencia 1/3(ReductionCte)
  minimum value1/1(min) -> Control de Temperatura1/2(Tq_RL), Control de Potencia 1/2(Tq_RL), else1/2(Tq_RL)
  Temperature_IGBT/1 -> If2/4
  Control de Potencia 1/2(Tq_RL_out) -> Merge4/1
  Power_limit1/1 -> If2/1

== system Torque_Control_ETR07/VDC/Vehicle Dynamics Control 2018/VDC 2018 without Longitudinal/Constraints/Braking with Regenerative ==
  MaxRegTorque : Inport
  Tq_RR_wc : Inport  Port=2
  Tq_RL_wc : Inport  Port=3
  Action Port : ActionPort  ActionType=then
  Gain : Gain  Gain=-1
  Gain1 : Gain  Gain=-1
  MATLAB Function : MATLAB Function  TreatAsAtomicUnit=on
  TQ_RR : Outport
  TQ_RL : Outport  Port=2
  wires:
  MATLAB Function/2(RegTq_RL) -> Gain1/1
  MATLAB Function/1(RegTq_RR) -> Gain/1
  Tq_RR_wc/1 -> MATLAB Function/2(Tq_RR)
  Tq_RL_wc/1 -> MATLAB Function/3(Tq_RL)
  MaxRegTorque/1 -> MATLAB Function/1(MaxRegenTq)
  Gain1/1 -> TQ_RL/1
  Gain/1 -> TQ_RR/1

== system Torque_Control_ETR07/VDC/Vehicle Dynamics Control 2018/VDC 2018 without Longitudinal/Driver // CarBehaviours/Accelerating ==
  Ap : Inport
  "Ap_Sat_up " : Inport  Port=2
  Ap_Sat_down : Inport  Port=3
  Tq_RR : Inport  Port=4
  "Tq_RL " : Inport  Port=5
  Action Port : ActionPort  ActionType=else
  "Accelerator behaviour " : MATLAB Function  TreatAsAtomicUnit=on
  Product : Product
  Product1 : Product
  "Tq_RR " : Outport
  Tq_RL : Outport  Port=2
  Out_Throttle : Outport  Port=3
  wires:
  Ap/1 -> "Accelerator behaviour "/1(Ap)
  "Ap_Sat_up "/1 -> "Accelerator behaviour "/2(Ap_Sat_up)
  Ap_Sat_down/1 -> "Accelerator behaviour "/3(Ap_Sat_down)
  Product1/1 -> "Tq_RR "/1
  Product/1 -> Tq_RL/1
  "Accelerator behaviour "/1(throttle) -> Out_Throttle/1, Product/1, Product1/1
  Tq_RR/1 -> Product1/2
  "Tq_RL "/1 -> Product/2

== system Torque_Control_ETR07/VDC/Vehicle Dynamics Control 2018/VDC 2018 without Longitudinal/Driver // CarBehaviours/Inertia Braking ==
  Action Port : ActionPort  ActionType=elseif
  Constant : Constant  Value=0
  Constant1 : Constant  Value=0
  "Tq_RR " : Outport
  Tq_RL : Outport  Port=2
  wires:
  Constant1/1 -> Tq_RL/1
  Constant/1 -> "Tq_RR "/1

== system Torque_Control_ETR07/VDC/Vehicle Dynamics Control 2018/VDC 2018 without Longitudinal/Driver // CarBehaviours/Mech_Braking ==
  Action Port : ActionPort  ActionType=elseif
  Constant : Constant  Value=0
  Constant1 : Constant  Value=0
  "Tq_RR " : Outport
  Tq_RL : Outport  Port=2
  wires:
  Constant1/1 -> Tq_RL/1
  Constant/1 -> "Tq_RR "/1

== system Torque_Control_ETR07/VDC/Vehicle Dynamics Control 2018/VDC 2018 without Longitudinal/Driver // CarBehaviours/Regenerative+Mech Braking ==
  RegTq_RR : Inport
  RegTq_RL : Inport  Port=2
  Action Port : ActionPort  ActionType=then
  "Tq_RR " : Outport
  Tq_RL : Outport  Port=2
  wires:
  RegTq_RL/1 -> Tq_RL/1
  RegTq_RR/1 -> "Tq_RR "/1

== system Torque_Control_ETR07/VDC/Vehicle Dynamics Control 2018/VDC 2018 without Longitudinal/Optimization SKF & CKF/Subsystem  ==
  Derivative : Inport
  "CKF_Initial " : Inport  Port=2
  "CKF_prev " : Inport  Port=3
  Cte_CKF : Inport  Port=4
  CKF : Subsystem
  CKF_act : Outport
  wires:
  CKF/1("CKF_act ") -> CKF_act/1
  "CKF_prev "/1 -> CKF/3("CKF_prev ")
  Derivative/1 -> CKF/1(Derivative)
  "CKF_Initial "/1 -> CKF/2(CKF_Initial)
  Cte_CKF/1 -> CKF/4(Cte_CKF)

== system Torque_Control_ETR07/VDC/Vehicle Dynamics Control 2018/VDC 2018 without Longitudinal/Wheel_to_engine/Fx_to_engineTqRL ==
  Fx : Inport
  Re : Inport  Port=2
  RT : Inport  Port=3
  Divide : Product  Inputs=*/
  Product : Product
  Tq : Outport
  wires:
  Divide/1 -> Tq/1
  Product/1 -> Divide/1
  RT/1 -> Divide/2
  Fx/1 -> Product/1
  Re/1 -> Product/2

== system Torque_Control_ETR07/VDC/Vehicle Dynamics Control 2018/VDC 2018 without Longitudinal/Wheel_to_engine/Fx_to_engineTqRR ==
  Fx : Inport
  Re : Inport  Port=2
  RT : Inport  Port=3
  Divide : Product  Inputs=*/
  Product : Product
  Tq : Outport
  wires:
  Divide/1 -> Tq/1
  Product/1 -> Divide/1
  RT/1 -> Divide/2
  Fx/1 -> Product/1
  Re/1 -> Product/2

== system Torque_Control_ETR07/VDC/Vehicle Dynamics Control 2018/Steering TV 2017 with TC/Optimization SKF & CKF/Subsystem /CKF ==
  Derivative : Inport
  CKF_Initial : Inport  Port=2
  "CKF_prev " : Inport  Port=3
  Cte_CKF : Inport  Port=4
  Action Port : ActionPort  ActionType=else
  If1 : If  IfExpression=u1 >= 900  ElseIfExpressions=u1 < 900  ShowElse=off
  Merge : Merge
  No spin : Subsystem  TreatAsAtomicUnit=on
  Saturation : Saturate  UpperLimit=1  LowerLimit=0.3
  "Spin " : Subsystem  TreatAsAtomicUnit=on
  "CKF_act " : Outport
  wires:
  Merge/1 -> Saturation/1
  "CKF_prev "/1 -> "Spin "/1(CKF_prev), No spin/2(CKF_prev)
  If1/1 -> "Spin "/Action
  Cte_CKF/1 -> "Spin "/3(Cte_CKF)
  "Spin "/1("CKF_act1 ") -> Merge/2
  Saturation/1 -> "CKF_act "/1
  CKF_Initial/1 -> "Spin "/2("CKF_Initial "), No spin/1(CKF_Initial)
  If1/2 -> No spin/Action
  No spin/1(CKF_act0) -> Merge/1
  Derivative/1 -> If1/1

== system Torque_Control_ETR07/VDC/Vehicle Dynamics Control 2018/Steering TV 2017 with TC/Optimization SKF & CKF/Subsystem /SKF ==
  Derivative : Inport
  "SKF_Initial " : Inport  Port=2
  SKF_prev : Inport  Port=3
  Cte_SKF : Inport  Port=4
  Action Port : ActionPort  ActionType=then
  Display : Display
  Display1 : Display
  If : If  IfExpression=u1 >=900  ElseIfExpressions=u1 < 900  ShowElse=off
  Merge : Merge
  No spin : Subsystem  TreatAsAtomicUnit=on
  Saturation : Saturate  UpperLimit=1  LowerLimit=0.3
  Spin : Subsystem  TreatAsAtomicUnit=on
  SKF_act : Outport
  wires:
  Merge/1 -> Saturation/1
  Spin/1(SKF_act1) -> Merge/2
  "SKF_Initial "/1 -> Spin/1(SKF_Initial), No spin/1(SKF_Initial)
  No spin/1(SKF_act0) -> Merge/1
  If/2 -> No spin/Action
  SKF_prev/1 -> Display/1, Spin/2(SKF_prev), No spin/2(SKF_prev)
  Cte_SKF/1 -> Spin/3(Cte_SKF)
  Saturation/1 -> Display1/1, SKF_act/1
  If/1 -> Spin/Action
  Derivative/1 -> If/1

== system Torque_Control_ETR07/VDC/Vehicle Dynamics Control 2018/VDC 2018 Complete/Constraints/Acelerating and braking without Regenerative/Control de Potencia  ==
  Tq_RR : Inport
  Tq_RL : Inport  Port=2
  ReductionCte : Inport  Port=3
  Action Port : ActionPort  ActionType=elseif
  Add : Sum  Inputs=+-
  Add1 : Sum  Inputs=+-
  Constant : Constant  Value=0
  Constant1 : Constant
  Product : Product
  Product1 : Product
  Tq_RR_out : Outport
  Tq_RL_out : Outport  Port=2
  Flag_Temperature : Outport  Port=3
  Flag_Power : Outport  Port=4
  wires:
  Tq_RR/1 -> Product/1, Add/1
  Tq_RL/1 -> Product1/1, Add1/1
  ReductionCte/1 -> Product/2, Product1/2
  Product1/1 -> Add1/2
  Product/1 -> Add/2
  Add1/1 -> Tq_RL_out/1
  Add/1 -> Tq_RR_out/1
  Constant1/1 -> Flag_Power/1
  Constant/1 -> Flag_Temperature/1

== system Torque_Control_ETR07/VDC/Vehicle Dynamics Control 2018/VDC 2018 Complete/Constraints/Acelerating and braking without Regenerative/Control de Temperatura ==
  Tq_RR : Inport
  Tq_RL : Inport  Port=2
  ReductionCte : Inport  Port=3
  Action Port : ActionPort  ActionType=then
  Add : Sum  Inputs=+-
  Add1 : Sum  Inputs=+-
  Constant : Constant
  Constant1 : Constant  Value=0
  Product : Product
  Product1 : Product
  Tq_RR_out : Outport
  Tq_RL_out : Outport  Port=2
  Flag_Temperature : Outport  Port=3
  Flag_Power : Outport  Port=4
  wires:
  Add/1 -> Tq_RR_out/1
  Add1/1 -> Tq_RL_out/1
  Product/1 -> Add/2
  Product1/1 -> Add1/2
  ReductionCte/1 -> Product1/2, Product/2
  Tq_RL/1 -> Add1/1, Product1/1
  Tq_RR/1 -> Add/1, Product/1
  Constant1/1 -> Flag_Power/1
  Constant/1 -> Flag_Temperature/1

== system Torque_Control_ETR07/VDC/Vehicle Dynamics Control 2018/VDC 2018 Complete/Constraints/Acelerating and braking without Regenerative/If Action 1 ==
  Trans_max_dynamic : Inport
  Action Port : ActionPort  ActionType=then
  Trans_limit : Outport
  wires:
  Trans_max_dynamic/1 -> Trans_limit/1

== system Torque_Control_ETR07/VDC/Vehicle Dynamics Control 2018/VDC 2018 Complete/Constraints/Acelerating and braking without Regenerative/If Action 2 ==
  "Trans_max_static " : Inport
  Action Port : ActionPort  ActionType=else
  Trans_limit : Outport
  wires:
  "Trans_max_static "/1 -> Trans_limit/1

== system Torque_Control_ETR07/VDC/Vehicle Dynamics Control 2018/VDC 2018 Complete/Constraints/Acelerating and braking without Regenerative/Momentum Z scaled ==
  Tq_RR_Lim : Inport
  Tq_RL_Lim : Inport  Port=2
  Tq_RR_wc : Inport  Port=3
  Tq_RL_wc : Inport  Port=4
  Tq_diff : Inport  Port=5
  Display : Display
  Display1 : Display
  MATLAB Function : MATLAB Function  TreatAsAtomicUnit=on
  TQ_RR : Outport
  TQ_RL : Outport  Port=2
  wires:
  Tq_RL_Lim/1 -> MATLAB Function/2(tq_RL_lim)
  Tq_RR_Lim/1 -> MATLAB Function/1(tq_RR_lim)
  Tq_RR_wc/1 -> MATLAB Function/3(tq_RR_wc)
  Tq_RL_wc/1 -> MATLAB Function/4(tq_RL_wc)
  MATLAB Function/1(TQ_RR) -> Display/1, TQ_RR/1
  MATLAB Function/2(TQ_RL) -> Display1/1, TQ_RL/1
  Tq_diff/1 -> MATLAB Function/5(tq_diff)
